simulink model "Lab05"  (R2024b)
settings: Solver=ode8  StartTime=0.0  StopTime=tf  FixedStep=0.025  RelTol=1e-3
values from neighbouring files (symbols this model uses):
  I = diag(Iv)    [initLab5.m]
  invI = inv(I)    [initLab5.m]
  w0 = [0.45; 0.52; 0.55]    [initLab5.m]
undefined symbols (not defined in the file or in its folder): IC
libraries: matrix_library x1
(part 1 of 4)
settings Model: Creator=elisa  LastModifiedBy=filippocamaleonte
settings ModelReferenceCC: ModelReferenceMinAlgLoopOccurrences=on
settings RTWCC: GPUComputeCapability=3.5

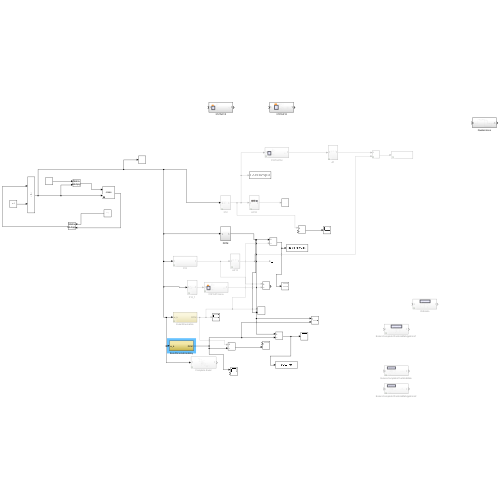
[thumbnail: Simulink's stored preview of the top-level diagram]
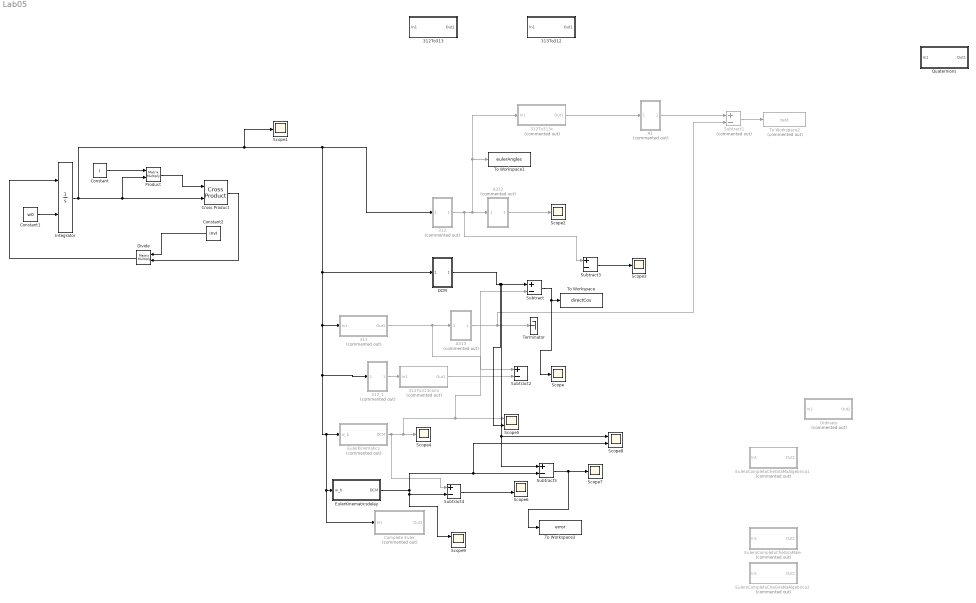
== system Lab05 ==
  312 : Subsystem  Commented=on
  312To313 : Subsystem
  312To313c : Subsystem  Commented=on
  312To313conv : Subsystem  Commented=on
  312_1 : Subsystem  Commented=on
  313 : Subsystem  Commented=on
  313To312 : Subsystem
  A1 : Subsystem  Commented=on
  A312 : Subsystem  Commented=on
  A313 : Subsystem  Commented=on
  Complete Euler : Subsystem  Commented=on
  Constant : Constant  Value=I
  Constant1 : Constant  Value=w0  VectorParams1D=off
  Constant2 : Constant  Value=invI
  Cross Product : matrix_library/Cross Product
  DCM : Subsystem
  Divide : Product  Inputs=**  Multiplication=Matrix(*)
  EulerKinematics : Subsystem  Commented=on
  EulerKinematicsdelay : Subsystem
  EuleroCompletoCheGiraMaAlgebrico1 : Subsystem  Commented=on
  EuleroCompletoCheGiraMaAlgebrico2 : Subsystem  Commented=on
  EuleroCompletoCheGiraMale : Subsystem  Commented=on
  Integrator : Integrator  InitialConditionSource=external
  Ordinato : Subsystem  Commented=on
  Product : Product  Multiplication=Matrix(*)
  Quaternions : Subsystem
  Scope{,1..4,7} (6 alike) : Scope
  Scope{5..6,8..9} (4 alike) : Scope  NumInputPorts=2
  Subtract{,2..5} (5 alike) : Sum  Inputs=+-
  Subtract1 : Sum  Commented=on  Inputs=+-
  Terminator : Terminator
  To Workspace : ToWorkspace  VariableName=directCos  SampleTime=-1
  To Workspace1 : ToWorkspace  VariableName=eulerAngles  SampleTime=-1
  To Workspace2 : ToWorkspace  Commented=on  VariableName=test  SampleTime=-1
  To Workspace3 : ToWorkspace  VariableName=error  SampleTime=-1
  wires:
  Product/1 -> Cross Product/1
  Cross Product/1 -> Divide/2
  Constant2/1 -> Divide/1
  Divide/1 -> Integrator/1
  Constant/1 -> Product/1
  Constant1/1 -> Integrator/2
  312/1(Out1) -> Subtract3/1, 312To313c/1(In1), To Workspace1/1, A312/1(In1)
  A313/1(Out1) -> Subtract1/2, Terminator/1
  Subtract/1 -> Scope/1, To Workspace/1
  A312/1(Out1) -> Scope2/1
  312To313c/1(Out1) -> A1/1(In1)
  A1/1(Out1) -> Subtract1/1
  Subtract1/1 -> To Workspace2/1
  312_1/1(Out1) -> 312To313conv/1(In1)
  312To313conv/1(Out1) -> Subtract2/2
  313/1(Out1) -> Subtract2/1, A313/1(In1)
  Subtract3/1 -> Scope3/1
  Integrator/1 -> Scope1/1, 313/1(In1), 312_1/1(In1), EulerKinematics/1(w_b), EulerKinematicsdelay/1(w_b), Complete Euler/1(In1), DCM/1(In1), 312/1(In1), Product/2, Cross Product/2
  EulerKinematics/1(DCM) -> Subtract4/1, Subtract/2, Scope5/1, Scope4/1
  DCM/1(Out1) -> Subtract/1, Scope8/1, Subtract5/1, Scope5/2
  Subtract4/1 -> Scope6/2
  EulerKinematicsdelay/1(DCM) -> Scope9/1, Subtract4/2, Scope8/2, Subtract5/2
  Subtract5/1 -> To Workspace3/1, Scope7/1

== system Lab05/312 ==
  In1 : Inport
  Cos1 : Trigonometry  Operator=cos
  Cos2 : Trigonometry  Operator=cos
  Demux : Demux  Outputs=3
  Divide1 : Product  Inputs=*/
  Integrator1 : Integrator  WrapState=on  WrappedStateUpperValue=2*pi  WrappedStateLowerValue=0
  Integrator2 : Integrator  InitialCondition=pi/4  WrapState=on
  Integrator3 : Integrator  WrapState=on  WrappedStateUpperValue=2*pi  WrappedStateLowerValue=0
  Mux : Mux  Inputs=3
  Product{1..7} (7 alike) : Product
  Sin : Trigonometry
  Subtract : Sum  Inputs=+-
  Subtract1 : Sum
  Subtract2 : Sum  Inputs=+-
  Subtract3 : Sum  Inputs=+-
  Tan : Trigonometry  Operator=tan
  Out1 : Outport
  wires:
  Product6/1 -> Subtract3/2
  Product5/1 -> Subtract3/1
  Product4/1 -> Subtract1/2
  Integrator3/1 -> [theta3]
  [wz] -> Product5/1
  Mux/1 -> Out1/1
  Product7/1 -> Subtract2/2
  Cos1/1 -> [cosPsi]
  [theta3] -> Sin/1, Cos1/1
  [cosPsi] -> Product1/2
  Demux/2 -> [wy]
  Tan/1 -> [tanThe]
  Product2/1 -> Subtract/2
  [wz] -> Product3/1
  [tanThe] -> Product7/2
  Cos2/1 -> [cosThe]
  [cosPsi] -> Product5/2
  Divide1/1 -> Integrator1/1
  Subtract1/1 -> Integrator2/1
  Demux/3 -> [wz]
  [theta1] -> Mux/1
  Subtract/1 -> Divide1/1
  Demux/1 -> [wx]
  Subtract2/1 -> Integrator3/1
  [theta2] -> Tan/1, Cos2/1
  [wy] -> Subtract2/1
  Integrator1/1 -> [theta1]
  Integrator2/1 -> [theta2]
  [wx] -> Product4/1
  [sinPsi] -> Product2/2
  In1/1 -> Demux/1
  Subtract3/1 -> Product7/1
  Product3/1 -> Subtract1/1
  [theta2] -> Mux/2
  [sinPsi] -> Product3/2
  [theta3] -> Mux/3
  [sinPsi] -> Product6/2
  [wx] -> Product6/1
  [wx] -> Product2/1
  [cosPsi] -> Product4/2
  [wz] -> Product1/1
  Product1/1 -> Subtract/1
  [cosThe] -> Divide1/2
  Sin/1 -> [sinPsi]

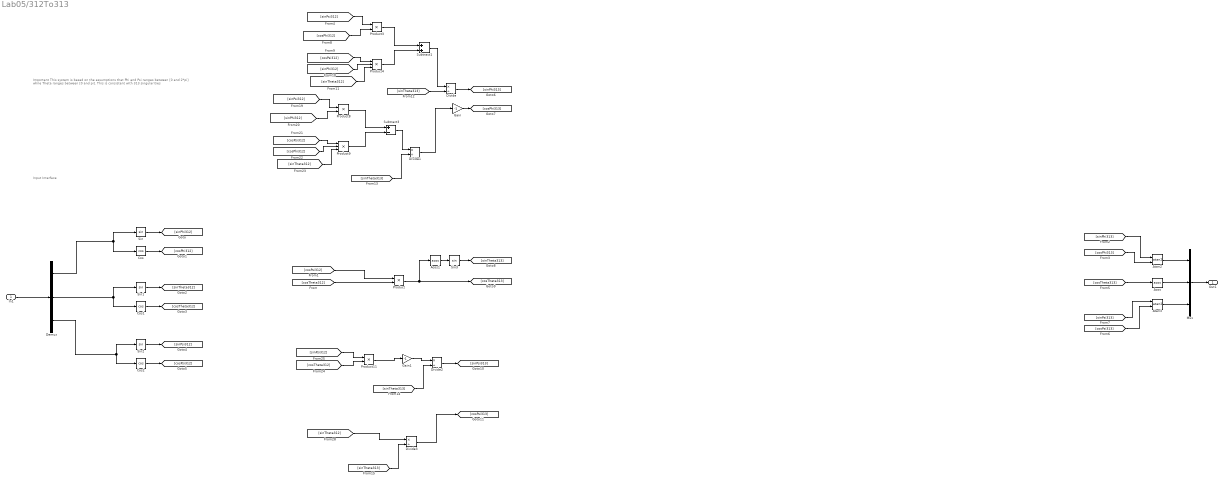
== system Lab05/312To313 ==
  note: Important
      |
      | This system is based on the assumptions that Phi and Psi ranges between [0 and 2*pi] while Theta ranges between [0 and pi]. This is consistent with 313 singularities
  note: Input Interface
  In1 : Inport
  Acos : Trigonometry  Operator=acos
  Acos1 : Trigonometry  Operator=acos
  Atan2 : Trigonometry  Operator=atan2
  Atan3 : Trigonometry  Operator=atan2
  Cos : Trigonometry  Operator=cos
  Cos1 : Trigonometry  Operator=cos
  Cos2 : Trigonometry  Operator=cos
  Demux : Demux  Outputs=3
  Divide{,1..3} (4 alike) : Product  Inputs=*/
  Gain : Gain  Gain=-1
  Gain1 : Gain  Gain=-1
  Mux : Mux  Inputs=3
  Product{,3,8,11} (4 alike) : Product
  Product4 : Product  Inputs=3
  Product9 : Product  Inputs=3
  Sin{,1..3} (4 alike) : Trigonometry
  Subtract1 : Sum
  Subtract3 : Sum  Inputs=+-
  Out1 : Outport
  wires:
  In1/1 -> Demux/1
  Mux/1 -> Out1/1
  Sin/1 -> [sinPhi312]
  Cos/1 -> [cosPhi312]
  Demux/1 -> Sin/1, Cos/1
  Sin1/1 -> [sinTheta312]
  Demux/2 -> Sin1/1, Cos1/1
  Cos1/1 -> [cosTheta312]
  Sin2/1 -> [sinPsi312]
  Cos2/1 -> [cosPsi312]
  Demux/3 -> Sin2/1, Cos2/1
  Product/1 -> Acos1/1, [cosTheta313]
  [cosTheta312] -> Product/2
  [cosPsi312] -> Product/1
  Atan2/1 -> Mux/1
  Acos/1 -> Mux/2
  Atan3/1 -> Mux/3
  [sinPhi313] -> Atan2/1
  [cosPhi313] -> Atan2/2
  [cosTheta313] -> Acos/1
  [cosPsi313] -> Atan3/2
  [sinPsi313] -> Atan3/1
  Sin3/1 -> [sinTheta313]
  Acos1/1 -> Sin3/1
  [cosPsi312] -> Product4/1
  [sinTheta312] -> Product4/3
  Product3/1 -> Subtract1/1
  [cosPhi312] -> Product3/2
  Product4/1 -> Subtract1/2
  [sinPsi312] -> Product3/1
  [sinPhi312] -> Product4/2
  Divide/1 -> [sinPhi313]
  [sinTheta313] -> Divide/2
  Subtract1/1 -> Divide/1
  Gain/1 -> [cosPhi313]
  Divide1/1 -> Gain/1
  [sinTheta313] -> Divide1/2
  [cosPsi312] -> Product9/1
  Product9/1 -> Subtract3/2
  Subtract3/1 -> Divide1/1
  [sinPsi312] -> Product8/1
  [cosPhi312] -> Product9/2
  [sinPhi312] -> Product8/2
  [sinTheta312] -> Product9/3
  Product8/1 -> Subtract3/1
  [sinTheta313] -> Divide2/2
  Divide2/1 -> [sinPsi313]
  [sinTheta313] -> Divide3/2
  Divide3/1 -> [cosPsi313]
  Product11/1 -> Gain1/1
  [sinPsi312] -> Product11/1
  [cosTheta312] -> Product11/2
  Gain1/1 -> Divide2/1
  [sinTheta312] -> Divide3/1

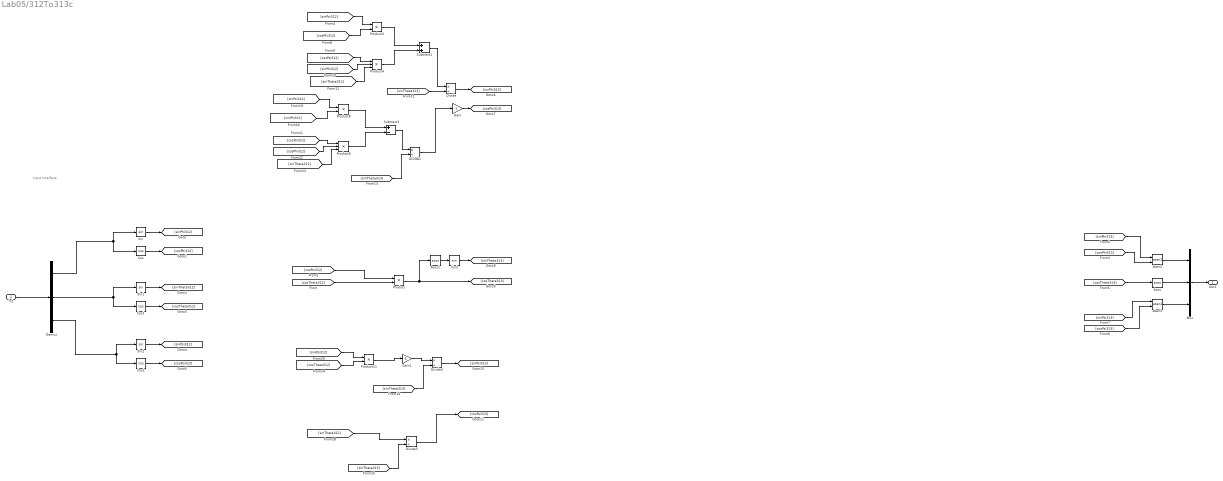
== system Lab05/312To313c ==
  note: Input Interface
  In1 : Inport
  Acos : Trigonometry  Operator=acos
  Acos1 : Trigonometry  Operator=acos
  Atan2 : Trigonometry  Operator=atan2
  Atan3 : Trigonometry  Operator=atan2
  Cos : Trigonometry  Operator=cos
  Cos1 : Trigonometry  Operator=cos
  Cos2 : Trigonometry  Operator=cos
  Demux : Demux  Outputs=3
  Divide{,1..3} (4 alike) : Product  Inputs=*/
  Gain : Gain  Gain=-1
  Gain1 : Gain  Gain=-1
  Mux : Mux  Inputs=3
  Product{,3,8,11} (4 alike) : Product
  Product4 : Product  Inputs=3
  Product9 : Product  Inputs=3
  Sin{,1..3} (4 alike) : Trigonometry
  Subtract1 : Sum
  Subtract3 : Sum  Inputs=+-
  Out1 : Outport
  wires:
  In1/1 -> Demux/1
  Mux/1 -> Out1/1
  Sin/1 -> [sinPhi312]
  Cos/1 -> [cosPhi312]
  Demux/1 -> Sin/1, Cos/1
  Sin1/1 -> [sinTheta312]
  Demux/2 -> Sin1/1, Cos1/1
  Cos1/1 -> [cosTheta312]
  Sin2/1 -> [sinPsi312]
  Cos2/1 -> [cosPsi312]
  Demux/3 -> Sin2/1, Cos2/1
  Product/1 -> Acos1/1, [cosTheta313]
  [cosTheta312] -> Product/2
  [cosPsi312] -> Product/1
  Atan2/1 -> Mux/1
  Acos/1 -> Mux/2
  Atan3/1 -> Mux/3
  [sinPhi313] -> Atan2/1
  [cosPhi313] -> Atan2/2
  [cosTheta313] -> Acos/1
  [cosPsi313] -> Atan3/2
  [sinPsi313] -> Atan3/1
  Sin3/1 -> [sinTheta313]
  Acos1/1 -> Sin3/1
  [cosPsi312] -> Product4/1
  [sinTheta312] -> Product4/3
  Product3/1 -> Subtract1/1
  [cosPhi312] -> Product3/2
  Product4/1 -> Subtract1/2
  [sinPsi312] -> Product3/1
  [sinPhi312] -> Product4/2
  Divide/1 -> [sinPhi313]
  [sinTheta313] -> Divide/2
  Subtract1/1 -> Divide/1
  Gain/1 -> [cosPhi313]
  Divide1/1 -> Gain/1
  [sinTheta313] -> Divide1/2
  [cosPsi312] -> Product9/1
  Product9/1 -> Subtract3/2
  Subtract3/1 -> Divide1/1
  [sinPsi312] -> Product8/1
  [cosPhi312] -> Product9/2
  [sinPhi312] -> Product8/2
  [sinTheta312] -> Product9/3
  Product8/1 -> Subtract3/1
  [sinTheta313] -> Divide2/2
  Divide2/1 -> [sinPsi313]
  [sinTheta313] -> Divide3/2
  Divide3/1 -> [cosPsi313]
  Product11/1 -> Gain1/1
  [sinPsi312] -> Product11/1
  [cosTheta312] -> Product11/2
  Gain1/1 -> Divide2/1
  [sinTheta312] -> Divide3/1

== system Lab05/312To313conv ==
  note: Important
      |
      | This system is based on the assumptions that Phi and Psi ranges between [0 and 2*pi] while Theta ranges between [0 and pi]. This is consistent with 313 singularities
  note: Input Interface
  In1 : Inport
  Acos : Trigonometry  Operator=acos
  Acos1 : Trigonometry  Operator=acos
  Atan2 : Trigonometry  Operator=atan2
  Atan3 : Trigonometry  Operator=atan2
  Cos : Trigonometry  Operator=cos
  Cos1 : Trigonometry  Operator=cos
  Cos2 : Trigonometry  Operator=cos
  Demux : Demux  Outputs=3
  Divide{,1..3} (4 alike) : Product  Inputs=*/
  Gain : Gain  Gain=-1
  Gain1 : Gain  Gain=-1
  Mux : Mux  Inputs=3
  Product{,3,8,11} (4 alike) : Product
  Product4 : Product  Inputs=3
  Product9 : Product  Inputs=3
  Sin{,1..3} (4 alike) : Trigonometry
  Subtract1 : Sum
  Subtract3 : Sum  Inputs=+-
  Out1 : Outport
  wires:
  In1/1 -> Demux/1
  Mux/1 -> Out1/1
  Sin/1 -> [sinPhi312]
  Cos/1 -> [cosPhi312]
  Demux/1 -> Sin/1, Cos/1
  Sin1/1 -> [sinTheta312]
  Demux/2 -> Sin1/1, Cos1/1
  Cos1/1 -> [cosTheta312]
  Sin2/1 -> [sinPsi312]
  Cos2/1 -> [cosPsi312]
  Demux/3 -> Sin2/1, Cos2/1
  Product/1 -> Acos1/1, [cosTheta313]
  [cosTheta312] -> Product/2
  [cosPsi312] -> Product/1
  Atan2/1 -> Mux/1
  Acos/1 -> Mux/2
  Atan3/1 -> Mux/3
  [sinPhi313] -> Atan2/1
  [cosPhi313] -> Atan2/2
  [cosTheta313] -> Acos/1
  [cosPsi313] -> Atan3/2
  [sinPsi313] -> Atan3/1
  Sin3/1 -> [sinTheta313]
  Acos1/1 -> Sin3/1
  [cosPsi312] -> Product4/1
  [sinTheta312] -> Product4/3
  Product3/1 -> Subtract1/1
  [cosPhi312] -> Product3/2
  Product4/1 -> Subtract1/2
  [sinPsi312] -> Product3/1
  [sinPhi312] -> Product4/2
  Divide/1 -> [sinPhi313]
  [sinTheta313] -> Divide/2
  Subtract1/1 -> Divide/1
  Gain/1 -> [cosPhi313]
  Divide1/1 -> Gain/1
  [sinTheta313] -> Divide1/2
  [cosPsi312] -> Product9/1
  Product9/1 -> Subtract3/2
  Subtract3/1 -> Divide1/1
  [sinPsi312] -> Product8/1
  [cosPhi312] -> Product9/2
  [sinPhi312] -> Product8/2
  [sinTheta312] -> Product9/3
  Product8/1 -> Subtract3/1
  [sinTheta313] -> Divide2/2
  Divide2/1 -> [sinPsi313]
  [sinTheta313] -> Divide3/2
  Divide3/1 -> [cosPsi313]
  Product11/1 -> Gain1/1
  [sinPsi312] -> Product11/1
  [cosTheta312] -> Product11/2
  Gain1/1 -> Divide2/1
  [sinTheta312] -> Divide3/1

== system Lab05/312_1 ==
  In1 : Inport
  Cos1 : Trigonometry  Operator=cos
  Cos2 : Trigonometry  Operator=cos
  Demux : Demux  Outputs=3
  Divide1 : Product  Inputs=*/
  Integrator1 : Integrator  WrapState=on  WrappedStateUpperValue=2*pi  WrappedStateLowerValue=0
  Integrator2 : Integrator  InitialCondition=pi/4  WrapState=on
  Integrator3 : Integrator  WrapState=on  WrappedStateUpperValue=2*pi  WrappedStateLowerValue=0
  Mux : Mux  Inputs=3
  Product{1..7} (7 alike) : Product
  Sin : Trigonometry
  Subtract : Sum  Inputs=+-
  Subtract1 : Sum
  Subtract2 : Sum  Inputs=+-
  Subtract3 : Sum  Inputs=+-
  Tan : Trigonometry  Operator=tan
  Out1 : Outport
  wires:
  Product6/1 -> Subtract3/2
  Product5/1 -> Subtract3/1
  Product4/1 -> Subtract1/2
  Integrator3/1 -> [theta3]
  [wz] -> Product5/1
  Mux/1 -> Out1/1
  Product7/1 -> Subtract2/2
  Cos1/1 -> [cosPsi]
  [theta3] -> Sin/1, Cos1/1
  [cosPsi] -> Product1/2
  Demux/2 -> [wy]
  Tan/1 -> [tanThe]
  Product2/1 -> Subtract/2
  [wz] -> Product3/1
  [tanThe] -> Product7/2
  Cos2/1 -> [cosThe]
  [cosPsi] -> Product5/2
  Divide1/1 -> Integrator1/1
  Subtract1/1 -> Integrator2/1
  Demux/3 -> [wz]
  [theta1] -> Mux/1
  Subtract/1 -> Divide1/1
  Demux/1 -> [wx]
  Subtract2/1 -> Integrator3/1
  [theta2] -> Tan/1, Cos2/1
  [wy] -> Subtract2/1
  Integrator1/1 -> [theta1]
  Integrator2/1 -> [theta2]
  [wx] -> Product4/1
  [sinPsi] -> Product2/2
  In1/1 -> Demux/1
  Subtract3/1 -> Product7/1
  Product3/1 -> Subtract1/1
  [theta2] -> Mux/2
  [sinPsi] -> Product3/2
  [theta3] -> Mux/3
  [sinPsi] -> Product6/2
  [wx] -> Product6/1
  [wx] -> Product2/1
  [cosPsi] -> Product4/2
  [wz] -> Product1/1
  Product1/1 -> Subtract/1
  [cosThe] -> Divide1/2
  Sin/1 -> [sinPsi]

== system Lab05/313 ==
  note: Phi
  note: Theta
  In1 : Inport
  Cos1 : Trigonometry  Operator=cos
  Cos2 : Trigonometry
  Demux : Demux  Outputs=3
  Divide : Product  Inputs=/
  Divide1 : Product  Inputs=*/
  Integrator1 : Integrator  WrapState=on  WrappedStateUpperValue=2*pi  WrappedStateLowerValue=0
  Integrator2 : Integrator  InitialCondition=pi/4  WrapState=on
  Integrator3 : Integrator  WrapState=on  WrappedStateUpperValue=2*pi  WrappedStateLowerValue=0
  Mux : Mux  Inputs=3
  Product{1..7} (7 alike) : Product
  Sin : Trigonometry
  Subtract : Sum
  Subtract1 : Sum  Inputs=-+
  Subtract2 : Sum  Inputs=+-
  Subtract3 : Sum
  Tan : Trigonometry  Operator=tan
  Out1 : Outport
  wires:
  [sinThe] -> Divide1/2
  Sin/1 -> [sinPsi]
  [wx] -> Product2/1
  [theta3] -> Mux/3
  [theta2] -> Mux/2
  Product3/1 -> Subtract1/1
  In1/1 -> Demux/1
  [sinPsi] -> Product3/2
  [sinPsi] -> Product6/2
  Subtract3/1 -> Product7/1
  Product1/1 -> Subtract/1
  [wx] -> Product6/1
  [wy] -> Product1/1
  [wz] -> Subtract2/1
  Subtract2/1 -> Integrator3/1
  [theta2] -> Tan/1, Cos2/1
  [cosPsi] -> Product4/2
  Demux/1 -> [wx]
  [sinPsi] -> Product2/2
  Integrator2/1 -> [theta2]
  [wx] -> Product4/1
  Tan/1 -> Divide/1
  [cosPsi] -> Product1/2
  Divide1/1 -> Integrator1/1
  Integrator1/1 -> [theta1]
  [ctanThe] -> Product7/2
  [cosPsi] -> Product5/2
  [wy] -> Product3/1
  Product2/1 -> Subtract/2
  Demux/2 -> [wy]
  Product5/1 -> Subtract3/1
  [wy] -> Product5/1
  Integrator3/1 -> [theta3]
  Product6/1 -> Subtract3/2
  Mux/1 -> Out1/1
  Product4/1 -> Subtract1/2
  [theta3] -> Sin/1, Cos1/1
  Product7/1 -> Subtract2/2
  Cos2/1 -> [sinThe]
  Subtract1/1 -> Integrator2/1
  [theta1] -> Mux/1
  Subtract/1 -> Divide1/1
  Demux/3 -> [wz]
  Cos1/1 -> [cosPsi]
  Divide/1 -> [ctanThe]

== system Lab05/313To312 ==
  note: Input Interface
  note: Important
      |
      | This system is based on the assumptions that Phi and Psi ranges between [0 and 2*pi] while Theta ranges between [-pi/2 and pi/2]. This is consistent with 312 singularities
  In1 : Inport
  Acos : Trigonometry  Operator=asin
  Acos1 : Trigonometry  Operator=asin
  Atan2 : Trigonometry  Operator=atan2
  Atan3 : Trigonometry  Operator=atan2
  Cos : Trigonometry  Operator=cos
  Cos1 : Trigonometry  Operator=cos
  Cos2 : Trigonometry  Operator=cos
  Demux : Demux  Outputs=3
  Divide{,1..3} (4 alike) : Product  Inputs=*/
  Gain : Gain  Gain=-1
  Gain1 : Gain  Gain=-1
  Mux : Mux  Inputs=3
  Product{,3,8,11} (4 alike) : Product
  Product4 : Product  Inputs=3
  Product9 : Product  Inputs=3
  Sin : Trigonometry
  Sin1 : Trigonometry
  Sin2 : Trigonometry
  Sin3 : Trigonometry  Operator=cos
  Subtract1 : Sum  Inputs=--
  Subtract3 : Sum  Inputs=-+
  Out1 : Outport
  wires:
  Cos/1 -> [cosPhi313]
  Sin/1 -> [sinPhi313]
  Cos1/1 -> [cosTheta313]
  Demux/3 -> Sin2/1, Cos2/1
  Demux/1 -> Sin/1, Cos/1
  Sin2/1 -> [sinPsi313]
  Sin1/1 -> [sinTheta313]
  In1/1 -> Demux/1
  Demux/2 -> Sin1/1, Cos1/1
  Cos2/1 -> [cosPsi313]
  Mux/1 -> Out1/1
  [sinTheta312] -> Acos/1
  Atan3/1 -> Mux/3
  Atan2/1 -> Mux/1
  [sinPhi312] -> Atan2/1
  [cosPhi312] -> Atan2/2
  [sinPsi312] -> Atan3/1
  [cosPsi312] -> Atan3/2
  Acos/1 -> Mux/2
  [sinTheta313] -> Product/2
  Product/1 -> Acos1/1, [sinTheta312]
  Sin3/1 -> [cosTheta312]
  [cosPsi313] -> Product/1
  Acos1/1 -> Sin3/1
  Gain/1 -> [sinPhi312]
  Divide/1 -> Gain/1
  [cosTheta312] -> Divide/2
  Product3/1 -> Subtract1/1
  [cosPhi313] -> Product3/2
  Product4/1 -> Subtract1/2
  [cosPsi313] -> Product4/1
  [sinPhi313] -> Product4/2
  Subtract1/1 -> Divide/1
  [sinPsi313] -> Product3/1
  [cosTheta313] -> Product4/3
  [cosTheta312] -> Divide1/2
  Divide1/1 -> [cosPhi312]
  [cosPsi313] -> Product9/1
  Product9/1 -> Subtract3/2
  [sinPsi313] -> Product8/1
  [sinPhi313] -> Product8/2
  Product8/1 -> Subtract3/1
  [cosTheta313] -> Product9/3
  Subtract3/1 -> Divide1/1
  [cosPhi313] -> Product9/2
  Divide2/1 -> Gain1/1
  [cosTheta312] -> Divide2/2
  Gain1/1 -> [sinPsi312]
  [sinTheta313] -> Product11/2
  Product11/1 -> Divide2/1
  [sinPsi313] -> Product11/1
  [cosTheta312] -> Divide3/2
  [cosTheta313] -> Divide3/1
  Divide3/1 -> [cosPsi312]

== system Lab05/A1 ==
  In1 : Inport
  Cos : Trigonometry  Operator=cos
  Cos1 : Trigonometry  Operator=cos
  Cos2 : Trigonometry  Operator=cos
  Demux : Demux  Outputs=3
  Gain : Gain  Gain=-1
  Matrix Concatenate : Concatenate  NumInputs=3  Mode=Multidimensional array
  Matrix Concatenate1 : Concatenate  NumInputs=3  Mode=Multidimensional array
  Matrix Concatenate3 : Concatenate  NumInputs=3  Mode=Multidimensional array  ConcatenateDimension=2
  Matrix Concatenate4 : Concatenate  NumInputs=3  Mode=Multidimensional array
  Product{1,3,5..6,8,10..12} (8 alike) : Product
  Product{2,4,7,9} (4 alike) : Product  Inputs=3
  Sin : Trigonometry
  Sin1 : Trigonometry
  Sin2 : Trigonometry
  Subtract : Sum  Inputs=+-
  Subtract1 : Sum  Inputs=--
  Subtract2 : Sum
  Subtract3 : Sum  Inputs=-+
  Out1 : Outport
  wires:
  In1/1 -> Demux/1
  [cosTheta] -> Product2/3
  Product7/1 -> Subtract2/2
  [sinTheta] -> Product11/2
  [sinPhi] -> Product8/2
  Sin/1 -> [sinPhi]
  [cosTheta] -> Product4/3
  [sinPhi] -> Product2/2
  [sinTheta] -> Product10/2
  Product5/1 -> Matrix Concatenate/3
  [cosPsi] -> Product6/1
  Demux/3 -> Sin2/1, Cos2/1
  Product9/1 -> Subtract3/2
  [cosTheta] -> Matrix Concatenate1/3
  Matrix Concatenate1/1 -> Matrix Concatenate3/3
  [sinPsi] -> Product11/1
  Product2/1 -> Subtract/2
  [sinPhi] -> Product4/2
  Subtract2/1 -> Matrix Concatenate4/1
  Matrix Concatenate4/1 -> Matrix Concatenate3/2
  [cosPsi] -> Product12/1
  Cos2/1 -> [cosPsi]
  Product10/1 -> Gain/1
  [sinPsi] -> Product2/1
  [sinPsi] -> Product8/1
  Sin2/1 -> [sinPsi]
  [cosTheta] -> Product7/3
  Subtract/1 -> Matrix Concatenate/1
  [cosPhi] -> Product10/1
  Subtract1/1 -> Matrix Concatenate/2
  Subtract3/1 -> Matrix Concatenate4/2
  Demux/2 -> Sin1/1, Cos1/1
  [cosTheta] -> Product9/3
  Product8/1 -> Subtract3/1
  [cosPhi] -> Product9/2
  [cosPsi] -> Product9/1
  Gain/1 -> Matrix Concatenate4/3
  [cosPsi] -> Product4/1
  Product11/1 -> Matrix Concatenate1/1
  Product1/1 -> Subtract/1
  [cosPhi] -> Product1/2
  [sinTheta] -> Product12/2
  [cosPhi] -> Product7/2
  [sinPhi] -> Product6/2
  Product6/1 -> Subtract2/1
  Demux/1 -> Sin/1, Cos/1
  [cosPsi] -> Product1/1
  [sinPsi] -> Product7/1
  Cos1/1 -> [cosTheta]
  Sin1/1 -> [sinTheta]
  [sinTheta] -> Product5/2
  [sinPsi] -> Product3/1
  Product12/1 -> Matrix Concatenate1/2
  [sinPhi] -> Product5/1
  Product3/1 -> Subtract1/1
  Product4/1 -> Subtract1/2
  [cosPhi] -> Product3/2
  Matrix Concatenate/1 -> Matrix Concatenate3/1
  Cos/1 -> [cosPhi]
  Matrix Concatenate3/1 -> Out1/1

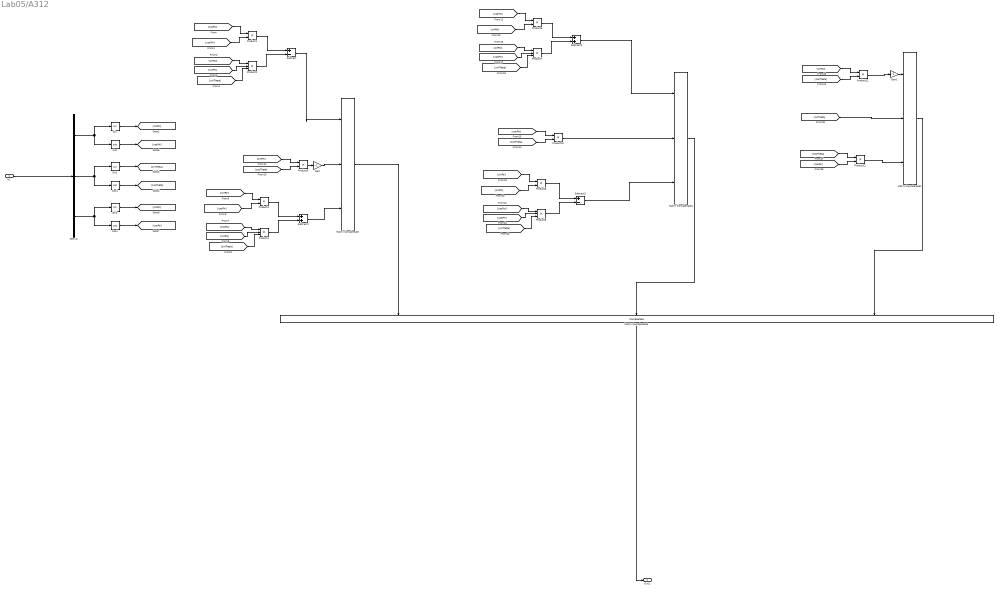
== system Lab05/A312 ==
  In1 : Inport
  Cos : Trigonometry  Operator=cos
  Cos1 : Trigonometry  Operator=cos
  Cos2 : Trigonometry  Operator=cos
  Demux : Demux  Outputs=3
  Gain : Gain  Gain=-1
  Gain1 : Gain  Gain=-1
  Matrix Concatenate : Concatenate  NumInputs=3  Mode=Multidimensional array
  Matrix Concatenate1 : Concatenate  NumInputs=3  Mode=Multidimensional array
  Matrix Concatenate3 : Concatenate  NumInputs=3  Mode=Multidimensional array  ConcatenateDimension=2
  Matrix Concatenate4 : Concatenate  NumInputs=3  Mode=Multidimensional array
  Product{1,3,5..6,8,10..12} (8 alike) : Product
  Product{2,4,7,9} (4 alike) : Product  Inputs=3
  Sin : Trigonometry
  Sin1 : Trigonometry
  Sin2 : Trigonometry
  Subtract : Sum  Inputs=+-
  Subtract1 : Sum
  Subtract2 : Sum
  Subtract3 : Sum  Inputs=+-
  Out1 : Outport
  wires:
  In1/1 -> Demux/1
  [sinTheta] -> Product2/3
  Product7/1 -> Subtract2/2
  [cosTheta] -> Product11/2
  [sinPhi] -> Product8/2
  Sin/1 -> [sinPhi]
  [sinPhi] -> Product2/2
  [cosTheta] -> Product10/2
  [cosPsi] -> Product6/1
  Demux/3 -> Sin2/1, Cos2/1
  Product9/1 -> Subtract3/2
  [sinTheta] -> Matrix Concatenate1/2
  Matrix Concatenate1/1 -> Matrix Concatenate3/3
  [sinPsi] -> Product11/1
  Product2/1 -> Subtract/2
  Subtract2/1 -> Matrix Concatenate4/1
  Matrix Concatenate4/1 -> Matrix Concatenate3/2
  [cosTheta] -> Product12/1
  Cos2/1 -> [cosPsi]
  [sinPsi] -> Product2/1
  [sinPsi] -> Product8/1
  Sin2/1 -> [sinPsi]
  [sinTheta] -> Product7/3
  Subtract/1 -> Matrix Concatenate/1
  [cosPhi] -> Product10/1
  Demux/2 -> Sin1/1, Cos1/1
  [sinTheta] -> Product9/3
  Product8/1 -> Subtract3/1
  [cosPhi] -> Product9/2
  [cosPsi] -> Product9/1
  Product11/1 -> Gain1/1
  Product1/1 -> Subtract/1
  [cosPhi] -> Product1/2
  [cosPsi] -> Product12/2
  [cosPhi] -> Product7/2
  [sinPhi] -> Product6/2
  Product6/1 -> Subtract2/1
  Demux/1 -> Sin/1, Cos/1
  [cosPsi] -> Product1/1
  [sinPsi] -> Product7/1
  Cos1/1 -> [cosTheta]
  Sin1/1 -> [sinTheta]
  Product12/1 -> Matrix Concatenate1/3
  Matrix Concatenate/1 -> Matrix Concatenate3/1
  Cos/1 -> [cosPhi]
  Matrix Concatenate3/1 -> Out1/1
  Gain1/1 -> Matrix Concatenate1/1
  Product10/1 -> Matrix Concatenate4/2
  Subtract3/1 -> Matrix Concatenate4/3
  [cosPsi] -> Product4/1
  Product4/1 -> Subtract1/2
  [cosPhi] -> Product3/2
  Product3/1 -> Subtract1/1
  [sinPsi] -> Product3/1
  [sinPhi] -> Product4/2
  [sinTheta] -> Product4/3
  [sinPhi] -> Product5/1
  [cosTheta] -> Product5/2
  Product5/1 -> Gain/1
  Subtract1/1 -> Matrix Concatenate/3
  Gain/1 -> Matrix Concatenate/2

== system Lab05/A313 ==
  In1 : Inport
  Cos : Trigonometry  Operator=cos
  Cos1 : Trigonometry  Operator=cos
  Cos2 : Trigonometry  Operator=cos
  Demux : Demux  Outputs=3
  Gain : Gain  Gain=-1
  Matrix Concatenate : Concatenate  NumInputs=3  Mode=Multidimensional array
  Matrix Concatenate1 : Concatenate  NumInputs=3  Mode=Multidimensional array
  Matrix Concatenate3 : Concatenate  NumInputs=3  Mode=Multidimensional array  ConcatenateDimension=2
  Matrix Concatenate4 : Concatenate  NumInputs=3  Mode=Multidimensional array
  Product{1,3,5..6,8,10..12} (8 alike) : Product
  Product{2,4,7,9} (4 alike) : Product  Inputs=3
  Sin : Trigonometry
  Sin1 : Trigonometry
  Sin2 : Trigonometry
  Subtract : Sum  Inputs=+-
  Subtract1 : Sum  Inputs=--
  Subtract2 : Sum
  Subtract3 : Sum  Inputs=-+
  Out1 : Outport
  wires:
  In1/1 -> Demux/1
  [cosTheta] -> Product2/3
  Product7/1 -> Subtract2/2
  [sinTheta] -> Product11/2
  [sinPhi] -> Product8/2
  Sin/1 -> [sinPhi]
  [cosTheta] -> Product4/3
  [sinPhi] -> Product2/2
  [sinTheta] -> Product10/2
  Product5/1 -> Matrix Concatenate/3
  [cosPsi] -> Product6/1
  Demux/3 -> Sin2/1, Cos2/1
  Product9/1 -> Subtract3/2
  [cosTheta] -> Matrix Concatenate1/3
  Matrix Concatenate1/1 -> Matrix Concatenate3/3
  [sinPsi] -> Product11/1
  Product2/1 -> Subtract/2
  [sinPhi] -> Product4/2
  Subtract2/1 -> Matrix Concatenate4/1
  Matrix Concatenate4/1 -> Matrix Concatenate3/2
  [cosPsi] -> Product12/1
  Cos2/1 -> [cosPsi]
  Product10/1 -> Gain/1
  [sinPsi] -> Product2/1
  [sinPsi] -> Product8/1
  Sin2/1 -> [sinPsi]
  [cosTheta] -> Product7/3
  Subtract/1 -> Matrix Concatenate/1
  [cosPhi] -> Product10/1
  Subtract1/1 -> Matrix Concatenate/2
  Subtract3/1 -> Matrix Concatenate4/2
  Demux/2 -> Sin1/1, Cos1/1
  [cosTheta] -> Product9/3
  Product8/1 -> Subtract3/1
  [cosPhi] -> Product9/2
  [cosPsi] -> Product9/1
  Gain/1 -> Matrix Concatenate4/3
  [cosPsi] -> Product4/1
  Product11/1 -> Matrix Concatenate1/1
  Product1/1 -> Subtract/1
  [cosPhi] -> Product1/2
  [sinTheta] -> Product12/2
  [cosPhi] -> Product7/2
  [sinPhi] -> Product6/2
  Product6/1 -> Subtract2/1
  Demux/1 -> Sin/1, Cos/1
  [cosPsi] -> Product1/1
  [sinPsi] -> Product7/1
  Cos1/1 -> [cosTheta]
  Sin1/1 -> [sinTheta]
  [sinTheta] -> Product5/2
  [sinPsi] -> Product3/1
  Product12/1 -> Matrix Concatenate1/2
  [sinPhi] -> Product5/1
  Product3/1 -> Subtract1/1
  Product4/1 -> Subtract1/2
  [cosPhi] -> Product3/2
  Matrix Concatenate/1 -> Matrix Concatenate3/1
  Cos/1 -> [cosPhi]
  Matrix Concatenate3/1 -> Out1/1

== system Lab05/Complete Euler ==
  In1 : Inport
  312 : Subsystem
  312To313 : Subsystem
  313 : Subsystem
  313To312 : Subsystem
  A312 : Subsystem
  A313 : Subsystem
  Abs : Abs  SaturateOnIntegerOverflow=off
  Abs1 : Abs  SaturateOnIntegerOverflow=off
  Constant : Constant
  Constant1 : Constant  Value=0
  Constant2 : Constant  Value=0
  Constant3 : Constant
  Cos : Trigonometry  Operator=cos
  Gain : Gain  Gain=-1
  Gain1 : Gain  Gain=-1
  Merge : Merge
  Selector : Selector  InputPortWidth=3  IndexOptions=Index vector (dialog)  Indices=[2]  OutputSizes=1
  Selector1 : Selector  InputPortWidth=3  IndexOptions=Index vector (dialog)  Indices=[2]  OutputSizes=1
  Sin : Trigonometry
  Switch : Switch  Criteria=u2 > Threshold  Threshold=-0.0001  SaturateOnIntegerOverflow=off  InputSameDT=off
  Switch1 : Switch  Criteria=u2 > Threshold  Threshold=-0.001  SaturateOnIntegerOverflow=off  InputSameDT=off
  Out1 : Outport
  wires:
  312To313/1(Out1) -> 313/2(In2)
  In1/1 -> 313/1(In1), 312/1(In1)
  313/1(Out1) -> 313To312/1(In1), Selector1/1, A313/1(In1)
  312/1(Out1) -> Selector/1, 312To313/1(In1), A312/1(In1)
  A313/1(Out1) -> Merge/2
  A312/1(Out1) -> Merge/1
  313To312/1(Out1) -> 312/2(In2)
  Selector/1 -> Cos/1
  Merge/1 -> Out1/1
  Cos/1 -> Abs/1
  Sin/1 -> Abs1/1
  Selector1/1 -> Sin/1
  Switch/1 -> 312/Enable
  Abs/1 -> Gain/1
  Switch1/1 -> 313/Enable
  Abs1/1 -> Gain1/1
  Constant/1 -> Switch1/1
  Gain/1 -> Switch1/2
  Gain1/1 -> Switch/2
  Constant1/1 -> Switch1/3
  Constant2/1 -> Switch/3
  Constant3/1 -> Switch/1

== system Lab05/DCM ==
  In1 : Inport
  A312 : Subsystem
  Constant3 : Constant  Value=IC.angles
  Gain : Gain  Gain=-1
  Integrator1 : Integrator  InitialConditionSource=external
  Product1 : Product  Multiplication=Matrix(*)
  Subsystem : Subsystem
  Subsystem1 : Subsystem
  w^ : Subsystem
  Out1 : Outport
  wires:
  w^/1(Out1) -> Gain/1
  Gain/1 -> Product1/1
  In1/1 -> w^/1(In1)
  Product1/1 -> Integrator1/1
  Constant3/1 -> A312/1(In1)
  Integrator1/1 -> Subsystem/1(In1)
  Subsystem/1(Out1) -> Subsystem1/1(In1)
  A312/1(Out1) -> Integrator1/2
  Subsystem1/1(Out1) -> Product1/2, Out1/1

== system Lab05/EulerKinematics ==
  note: Logic
  note: The flag is set to -1 when 313 is used and to 1 when 312 is used
  w_b : Inport
  312 Propagator : Subsystem
  312To313 : Subsystem
  313 Propagator : Subsystem
  313To312 : Subsystem
  A312 : Subsystem
  A313 : Subsystem
  Abs : Abs  SaturateOnIntegerOverflow=off
  Cos : Trigonometry  Operator=cos
  IC : InitialCondition  Value=IC.angles
  IC1 : InitialCondition  Value=IC.angles
  IC3 : InitialCondition
  Relay : Relay  OnSwitchValue=0.85  OffSwitchValue=0.15  OffOutputValue=-1
  Selector1 : Selector  InputPortWidth=3  IndexOptions=Index vector (dialog)  Indices=[2]  OutputSizes=1
  Switch : Switch  Criteria=u2 > Threshold  SaturateOnIntegerOverflow=off  InputSameDT=off
  Switch1 : Switch  Criteria=u2 > Threshold  SaturateOnIntegerOverflow=off  InputSameDT=off
  To Workspace : ToWorkspace  VariableName=flag  SampleTime=-1
  DCM : Outport
  wires:
  [EulerFlag] -> Switch1/2
  Cos/1 -> Abs/1
  Selector1/1 -> Cos/1
  Abs/1 -> Relay/1
  A313/1(Out1) -> Switch/3
  [Euler313] -> Switch1/3
  w_b/1 -> 313 Propagator/2(w_b), 312 Propagator/2(w_b)  "w_b"
  313 Propagator/1(EA) -> A313/1(Euler Angles), [Euler313]  "EulerAngles313"
  [Euler312] -> Switch1/1
  A312/1(DCM) -> Switch/1
  Switch1/1 -> Selector1/1
  Switch/1 -> DCM/1  "DCM"
  Relay/1 -> IC3/1
  IC3/1 -> To Workspace/1, [EulerFlag]
  313To312/1(Out1) -> IC1/1
  312To313/1(Out1) -> IC/1
  [Euler313] -> 313To312/1(In1)
  IC1/1 -> 312 Propagator/1(IC)
  IC/1 -> 313 Propagator/3(IC)
  [Euler312] -> 312To313/1(In1)
  [EulerFlag] -> Switch/2, 312 Propagator/3(Reset), 313 Propagator/1(Reset)
  312 Propagator/1(EA) -> [Euler312], A312/1(Euler Angles)  "EulerAngles312"

== system Lab05/EulerKinematicsdelay ==
  note: Logic
  note: The flag is set to -1 when 313 is used and to 1 when 312 is used
  w_b : Inport
  312 Propagator : Subsystem
  312To313 : Subsystem
  313 Propagator : Subsystem
  313To312 : Subsystem
  A312 : Subsystem
  A313 : Subsystem
  Abs : Abs  SaturateOnIntegerOverflow=off
  Cos : Trigonometry  Operator=cos
  IC : InitialCondition  Value=IC.angles
  IC1 : InitialCondition  Value=IC.angles
  IC3 : InitialCondition
  Relay : Relay  OnSwitchValue=0.75  OffSwitchValue=0.35  OffOutputValue=-1
  Selector1 : Selector  InputPortWidth=3  IndexOptions=Index vector (dialog)  Indices=[2]  OutputSizes=1
  Switch : Switch  Criteria=u2 > Threshold  SaturateOnIntegerOverflow=off  InputSameDT=off
  Switch1 : Switch  Criteria=u2 > Threshold  SaturateOnIntegerOverflow=off  InputSameDT=off
  To Workspace : ToWorkspace  VariableName=flag1  SampleTime=-1
  To Workspace1 : ToWorkspace  VariableName=eu312  SampleTime=-1
  To Workspace2 : ToWorkspace  VariableName=eu313  SampleTime=-1
  DCM : Outport
  wires:
  Cos/1 -> Abs/1
  Selector1/1 -> Cos/1
  Abs/1 -> Relay/1
  A313/1(Out1) -> Switch/3
  w_b/1 -> 313 Propagator/2(w_b), 312 Propagator/2(w_b)  "w_b"
  313 Propagator/1(EA) -> [Euler313], A313/1(Euler Angles)  "EulerAngles313"
  A312/1(DCM) -> Switch/1
  Switch1/1 -> Selector1/1
  Switch/1 -> DCM/1  "DCM"
  313To312/1(Out1) -> IC1/1
  312To313/1(Out1) -> IC/1
  IC1/1 -> 312 Propagator/1(IC)
  IC/1 -> 313 Propagator/3(IC)
  [EulerFlag] -> Switch/2, 312 Propagator/3(Reset), 313 Propagator/1(Reset)
  312 Propagator/1(EA) -> [Euler312], A312/1(Euler Angles)  "EulerAngles312"
  312 Propagator/2(Out1) -> 312To313/1(In1)
  313 Propagator/2(Out1) -> 313To312/1(In1)
  Relay/1 -> IC3/1
  [Euler312] -> To Workspace1/1, Switch1/1
  [Euler313] -> To Workspace2/1, Switch1/3
  [EulerFlag] -> Switch1/2
  IC3/1 -> To Workspace/1, [EulerFlag]

== system Lab05/EuleroCompletoCheGiraMaAlgebrico1 ==
  note: Logic
  note: The flag is set to -1 when 313 is used and to 1 when 312 is used
  In1 : Inport
  312 : Subsystem
  312To313 : Subsystem
  313 : Subsystem
  313To312 : Subsystem
  A312 : Subsystem
  A313 : Subsystem
  Abs : Abs  SaturateOnIntegerOverflow=off
  Cos : Trigonometry  Operator=cos
  IC : InitialCondition  Value=IC.angles
  IC1 : InitialCondition  Value=IC.angles
  IC3 : InitialCondition
  Relay : Relay  OnSwitchValue=0.7  OffSwitchValue=0.2  OffOutputValue=-1
  Selector1 : Selector  InputPortWidth=3  IndexOptions=Index vector (dialog)  Indices=[2]  OutputSizes=1
  Switch : Switch  Criteria=u2 > Threshold  SaturateOnIntegerOverflow=off  InputSameDT=off
  Switch1 : Switch  Criteria=u2 > Threshold  SaturateOnIntegerOverflow=off  InputSameDT=off
  To Workspace : ToWorkspace  VariableName=flag  SampleTime=-1
  Out1 : Outport
  wires:
  Switch/1 -> Out1/1
  Abs/1 -> Relay/1
  Cos/1 -> Abs/1
  [EulerFlag] -> 312/3(In3), Switch/2, 313/1(In3)
  A312/1(Out1) -> Switch/1
  A313/1(Out1) -> Switch/3
  Switch1/1 -> Selector1/1
  In1/1 -> 313/2(In1), 312/2(In1)
  [Euler313] -> Switch1/3
  [Euler312] -> Switch1/1
  Selector1/1 -> Cos/1
  [EulerFlag] -> Switch1/2
  IC3/1 -> To Workspace/1, [EulerFlag]
  Relay/1 -> IC3/1
  [Euler313] -> 313To312/1(In1)
  312/1(Out1) -> A312/1(In1), [Euler312]
  313/1(Out1) -> A313/1(In1), [Euler313]
  [Euler312] -> IC/1
  313To312/1(Out1) -> IC1/1
  312To313/1(Out1) -> 313/3(In2)
  IC/1 -> 312To313/1(In1)
  IC1/1 -> 312/1(In2)

== system Lab05/EuleroCompletoCheGiraMaAlgebrico2 ==
  note: Logic
  note: The flag is set to -1 when 313 is used and to 1 when 312 is used
  In1 : Inport
  312 : Subsystem
  312To313 : Subsystem
  313 : Subsystem
  313To1 : Subsystem
  313To312 : Subsystem
  A312 : Subsystem
  A313 : Subsystem
  Abs : Abs  SaturateOnIntegerOverflow=off
  Cos : Trigonometry  Operator=cos
  Gain : Gain  Gain=-1
  IC3 : InitialCondition
  Relay : Relay  OnSwitchValue=0.8  OffSwitchValue=0.2  OffOutputValue=-1
  Scope : Scope
  Scope1 : Scope
  Scope2 : Scope
  Selector1 : Selector  InputPortWidth=3  IndexOptions=Index vector (dialog)  Indices=[2]  OutputSizes=1
  Subtract : Sum  Inputs=+-
  Subtract1 : Sum  Inputs=+-
  Switch : Switch  Criteria=u2 > Threshold  SaturateOnIntegerOverflow=off  InputSameDT=off
  Switch1 : Switch  Criteria=u2 > Threshold  SaturateOnIntegerOverflow=off  InputSameDT=off
  To Workspace : ToWorkspace  VariableName=flag  SampleTime=-1
  Out1 : Outport
  wires:
  Switch/1 -> Out1/1
  Abs/1 -> Relay/1
  Cos/1 -> Abs/1
  [EulerFlag] -> Gain/1, Switch/2, 313/3(In3)
  A312/1(Out1) -> Switch/1, Scope2/1, Subtract1/1
  A313/1(Out1) -> Subtract1/2, Switch/3
  Switch1/1 -> Selector1/1
  In1/1 -> 313/2(In1), 312/1(In1)
  [EulerFlag] -> 312/3(In3)
  313To312/1(Out1) -> 312/2(In2)
  312To313/1(Out1) -> 313/1(In2)
  [Euler313] -> Switch1/3
  [Euler312] -> Switch1/1
  Selector1/1 -> Cos/1
  [EulerFlag] -> Switch1/2
  IC3/1 -> To Workspace/1, [EulerFlag]
  [Euler312] -> Subtract/2
  Subtract/1 -> Scope/1
  Relay/1 -> IC3/1
  [Euler313] -> 313To1/1(In1)
  313To1/1(Out1) -> Subtract/1
  Subtract1/1 -> Scope1/1
  [Euler312] -> 312To313/1(In1)
  [Euler313] -> 313To312/1(In1)
  312/1(Out1) -> [Euler312], A312/1(In1)
  313/1(Out1) -> A313/1(In1), [Euler313]

== system Lab05/EuleroCompletoCheGiraMale ==
  note: Logic
  note: The flag is set to -1 when 313 is used and to 1 when 312 is used
  In1 : Inport
  312 : Subsystem
  312To313 : Subsystem
  313 : Subsystem
  313To1 : Subsystem
  313To312 : Subsystem
  A312 : Subsystem
  A313 : Subsystem
  Abs : Abs  SaturateOnIntegerOverflow=off
  Cos : Trigonometry  Operator=cos
  Gain : Gain  Gain=-1
  IC : InitialCondition
  IC1 : InitialCondition  Value=IC.angles
  IC2 : InitialCondition  Value=IC.angles
  IC3 : InitialCondition
  Relay : Relay  OnSwitchValue=0.80  OffSwitchValue=0.2  OffOutputValue=-1
  Scope : Scope
  Scope1 : Scope
  Selector1 : Selector  InputPortWidth=3  IndexOptions=Index vector (dialog)  Indices=[2]  OutputSizes=1
  Subtract : Sum  Inputs=+-
  Subtract1 : Sum  Inputs=+-
  Switch : Switch  Criteria=u2 > Threshold  SaturateOnIntegerOverflow=off  InputSameDT=off
  Switch1 : Switch  Criteria=u2 > Threshold  SaturateOnIntegerOverflow=off  InputSameDT=off
  To Workspace : ToWorkspace  VariableName=flag  SaveFormat=Timeseries  SampleTime=-1
  Unit Delay : UnitDelay  SampleTime=-1  HasFrameUpgradeWarning=on
  Unit Delay1 : UnitDelay  SampleTime=-1  HasFrameUpgradeWarning=on
  Unit Delay2 : UnitDelay  SampleTime=-1  HasFrameUpgradeWarning=on
  Out1 : Outport
  wires:
  Switch/1 -> Out1/1
  Abs/1 -> Relay/1
  Cos/1 -> Abs/1
  [EulerFlag] -> Gain/1, Switch/2
  312/1(Out1) -> IC2/1
  A312/1(Out1) -> Subtract1/1, Switch/1
  313/1(Out1) -> IC1/1
  A313/1(Out1) -> Subtract1/2, Switch/3
  Switch1/1 -> Selector1/1
  [EulerFlag] -> IC/1
  In1/1 -> 313/2(In1), 312/1(In1)
  [EulerFlag] -> 312/Enable
  Gain/1 -> 313/Enable
  313To312/1(Out1) -> 312/2(In2)
  312To313/1(Out1) -> 313/1(In2)
  [Euler312] -> Unit Delay2/1
  [Euler313] -> Unit Delay1/1
  [Euler313] -> Switch1/3
  [Euler312] -> Switch1/1
  Selector1/1 -> Cos/1
  IC1/1 -> A313/1(In1), [Euler313]
  IC2/1 -> [Euler312], A312/1(In1)
  IC/1 -> Switch1/2
  IC3/1 -> To Workspace/1, [EulerFlag]
  [Euler312] -> Subtract/2
  Subtract/1 -> Scope/1
  Unit Delay/1 -> IC3/1
  Relay/1 -> Unit Delay/1
  Unit Delay1/1 -> 313To312/1(In1)
  [Euler313] -> 313To1/1(In1)
  313To1/1(Out1) -> Subtract/1
  Subtract1/1 -> Scope1/1
  Unit Delay2/1 -> 312To313/1(In1)

== system Lab05/Ordinato ==
  note: Logic
  note: The flag is set to -1 when 313 is used and to 1 when 312 is used
  In2 : Inport
  312 : Subsystem
  312To313 : Subsystem
  313 : Subsystem
  313To312 : Subsystem
  A312 : Subsystem
  A313 : Subsystem
  Abs : Abs  SaturateOnIntegerOverflow=off
  Cos : Trigonometry  Operator=cos
  IC : InitialCondition  Value=IC.angles
  IC1 : InitialCondition  Value=IC.angles
  IC3 : InitialCondition
  Relay : Relay  OnSwitchValue=0.65  OffSwitchValue=0.35  OffOutputValue=-1
  Selector1 : Selector  InputPortWidth=3  IndexOptions=Index vector (dialog)  Indices=[2]  OutputSizes=1
  Switch : Switch  Criteria=u2 > Threshold  SaturateOnIntegerOverflow=off  InputSameDT=off
  Switch1 : Switch  Criteria=u2 > Threshold  SaturateOnIntegerOverflow=off  InputSameDT=off
  To Workspace : ToWorkspace  VariableName=flag  SampleTime=-1
  Out2 : Outport
  wires:
  [EulerFlag] -> Switch1/2
  Cos/1 -> Abs/1
  Selector1/1 -> Cos/1
  Abs/1 -> Relay/1
  A313/1(Out1) -> Switch/3
  [Euler313] -> Switch1/3
  In2/1 -> 313/2(In1), 312/2(In1)
  313/1(Out1) -> A313/1(In1), [Euler313]
  [Euler312] -> Switch1/1
  A312/1(Out1) -> Switch/1
  Switch1/1 -> Selector1/1
  Switch/1 -> Out2/1
  Relay/1 -> IC3/1
  IC3/1 -> To Workspace/1, [EulerFlag]
  313To312/1(Out1) -> IC1/1
  312To313/1(Out1) -> IC/1
  [Euler313] -> 313To312/1(In1)
  IC1/1 -> 312/1(In2)
  IC/1 -> 313/3(In2)
  [Euler312] -> 312To313/1(In1)
  [EulerFlag] -> Switch/2, 312/3(In3), 313/1(In3)
  312/1(Out1) -> [Euler312], A312/1(In1)

== system Lab05/Quaternions ==
  In1 : Inport
  Gain : Gain  Gain=0.5  Multiplication=Matrix(u*K)
  Integrator : Integrator
  Matrix Multiply : Product  Multiplication=Matrix(*)
  Omega : Subsystem
  Out1 : Outport
  wires:
  Integrator/1 -> Matrix Multiply/2, Out1/1
  In1/1 -> Omega/1(In1)
  Omega/1(Out1) -> Gain/1
  Gain/1 -> Matrix Multiply/1
  Matrix Multiply/1 -> Integrator/1

== system Lab05/Complete Euler/312 ==
  In1 : Inport
  In2 : Inport  Port=2
  Enable : EnablePort  StatesWhenEnabling=reset
  Cos1 : Trigonometry  Operator=cos
  Cos2 : Trigonometry  Operator=cos
  Demux : Demux  Outputs=3
  Demux1 : Demux  Outputs=3
  Divide1 : Product  Inputs=*/
  IC : InitialCondition  Value=IC.angles
  Integrator1 : Integrator  InitialConditionSource=external  WrapState=on  WrappedStateUpperValue=2*pi  WrappedStateLowerValue=0
  Integrator2 : Integrator  InitialConditionSource=external  WrapState=on
  Integrator3 : Integrator  InitialConditionSource=external  WrapState=on  WrappedStateUpperValue=2*pi  WrappedStateLowerValue=0
  Mux : Mux  Inputs=3
  Product{1..7} (7 alike) : Product
  Sin : Trigonometry
  Subtract : Sum  Inputs=+-
  Subtract1 : Sum
  Subtract2 : Sum  Inputs=+-
  Subtract3 : Sum  Inputs=+-
  Tan : Trigonometry  Operator=tan
  Out1 : Outport
  wires:
  Product6/1 -> Subtract3/2
  Product5/1 -> Subtract3/1
  Product4/1 -> Subtract1/2
  Integrator3/1 -> [theta3]
  [wz] -> Product5/1
  Mux/1 -> Out1/1
  Product7/1 -> Subtract2/2
  Cos1/1 -> [cosPsi]
  [theta3] -> Sin/1, Cos1/1
  [cosPsi] -> Product1/2
  Demux/2 -> [wy]
  Tan/1 -> [tanThe]
  Product2/1 -> Subtract/2
  [wz] -> Product3/1
  [tanThe] -> Product7/2
  Cos2/1 -> [cosThe]
  [cosPsi] -> Product5/2
  Divide1/1 -> Integrator1/1
  Subtract1/1 -> Integrator2/1
  Demux/3 -> [wz]
  [theta1] -> Mux/1
  Subtract/1 -> Divide1/1
  Demux/1 -> [wx]
  Subtract2/1 -> Integrator3/1
  [theta2] -> Tan/1, Cos2/1
  [wy] -> Subtract2/1
  Integrator1/1 -> [theta1]
  Integrator2/1 -> [theta2]
  [wx] -> Product4/1
  [sinPsi] -> Product2/2
  In1/1 -> Demux/1
  Subtract3/1 -> Product7/1
  Product3/1 -> Subtract1/1
  [theta2] -> Mux/2
  [sinPsi] -> Product3/2
  [theta3] -> Mux/3
  [sinPsi] -> Product6/2
  [wx] -> Product6/1
  [wx] -> Product2/1
  [cosPsi] -> Product4/2
  [wz] -> Product1/1
  Product1/1 -> Subtract/1
  [cosThe] -> Divide1/2
  Sin/1 -> [sinPsi]
  Demux1/1 -> Integrator1/2
  Demux1/2 -> Integrator2/2
  Demux1/3 -> Integrator3/2
  In2/1 -> IC/1
  IC/1 -> Demux1/1

== system Lab05/Complete Euler/312To313 ==
  note: Important
      |
      | This system is based on the assumptions that Phi and Psi ranges between [0 and 2*pi] while Theta ranges between [0 and pi]. This is consistent with 313 singularities
  note: Input Interface
  In1 : Inport
  Acos : Trigonometry  Operator=acos
  Acos1 : Trigonometry  Operator=acos
  Atan2 : Trigonometry  Operator=atan2
  Atan3 : Trigonometry  Operator=atan2
  Cos : Trigonometry  Operator=cos
  Cos1 : Trigonometry  Operator=cos
  Cos2 : Trigonometry  Operator=cos
  Demux : Demux  Outputs=3
  Divide{,1..3} (4 alike) : Product  Inputs=*/
  Gain : Gain  Gain=-1
  Gain1 : Gain  Gain=-1
  Mux : Mux  Inputs=3
  Product{,3,8,11} (4 alike) : Product
  Product4 : Product  Inputs=3
  Product9 : Product  Inputs=3
  Sin{,1..3} (4 alike) : Trigonometry
  Subtract1 : Sum
  Subtract3 : Sum  Inputs=+-
  Out1 : Outport
  wires:
  In1/1 -> Demux/1
  Mux/1 -> Out1/1
  Sin/1 -> [sinPhi312]
  Cos/1 -> [cosPhi312]
  Demux/1 -> Sin/1, Cos/1
  Sin1/1 -> [sinTheta312]
  Demux/2 -> Sin1/1, Cos1/1
  Cos1/1 -> [cosTheta312]
  Sin2/1 -> [sinPsi312]
  Cos2/1 -> [cosPsi312]
  Demux/3 -> Sin2/1, Cos2/1
  Product/1 -> Acos1/1, [cosTheta313]
  [cosTheta312] -> Product/2
  [cosPsi312] -> Product/1
  Atan2/1 -> Mux/1
  Acos/1 -> Mux/2
  Atan3/1 -> Mux/3
  [sinPhi313] -> Atan2/1
  [cosPhi313] -> Atan2/2
  [cosTheta313] -> Acos/1
  [cosPsi313] -> Atan3/2
  [sinPsi313] -> Atan3/1
  Sin3/1 -> [sinTheta313]
  Acos1/1 -> Sin3/1
  [cosPsi312] -> Product4/1
  [sinTheta312] -> Product4/3
  Product3/1 -> Subtract1/1
  [cosPhi312] -> Product3/2
  Product4/1 -> Subtract1/2
  [sinPsi312] -> Product3/1
  [sinPhi312] -> Product4/2
  Divide/1 -> [sinPhi313]
  [sinTheta313] -> Divide/2
  Subtract1/1 -> Divide/1
  Gain/1 -> [cosPhi313]
  Divide1/1 -> Gain/1
  [sinTheta313] -> Divide1/2
  [cosPsi312] -> Product9/1
  Product9/1 -> Subtract3/2
  Subtract3/1 -> Divide1/1
  [sinPsi312] -> Product8/1
  [cosPhi312] -> Product9/2
  [sinPhi312] -> Product8/2
  [sinTheta312] -> Product9/3
  Product8/1 -> Subtract3/1
  [sinTheta313] -> Divide2/2
  Divide2/1 -> [sinPsi313]
  [sinTheta313] -> Divide3/2
  Divide3/1 -> [cosPsi313]
  Product11/1 -> Gain1/1
  [sinPsi312] -> Product11/1
  [cosTheta312] -> Product11/2
  Gain1/1 -> Divide2/1
  [sinTheta312] -> Divide3/1

== system Lab05/Complete Euler/313 ==
  note: Phi
  note: Theta
  In1 : Inport
  In2 : Inport  Port=2
  Enable : EnablePort  StatesWhenEnabling=reset
  Cos1 : Trigonometry  Operator=cos
  Cos2 : Trigonometry
  Demux : Demux  Outputs=3
  Demux1 : Demux  Outputs=3
  Divide : Product  Inputs=/
  Divide1 : Product  Inputs=*/
  IC : InitialCondition  Value=IC.angles
  Integrator1 : Integrator  InitialConditionSource=external  WrapState=on  WrappedStateUpperValue=2*pi  WrappedStateLowerValue=0
  Integrator2 : Integrator  InitialConditionSource=external  InitialCondition=pi/4  WrapState=on
  Integrator3 : Integrator  InitialConditionSource=external  WrapState=on  WrappedStateUpperValue=2*pi  WrappedStateLowerValue=0
  Mux : Mux  Inputs=3
  Product{1..7} (7 alike) : Product
  Sin : Trigonometry
  Subtract : Sum
  Subtract1 : Sum  Inputs=-+
  Subtract2 : Sum  Inputs=+-
  Subtract3 : Sum
  Tan : Trigonometry  Operator=tan
  Out1 : Outport
  wires:
  [sinThe] -> Divide1/2
  Sin/1 -> [sinPsi]
  [wx] -> Product2/1
  [theta3] -> Mux/3
  [theta2] -> Mux/2
  Product3/1 -> Subtract1/1
  In1/1 -> Demux/1
  [sinPsi] -> Product3/2
  [sinPsi] -> Product6/2
  Subtract3/1 -> Product7/1
  Product1/1 -> Subtract/1
  [wx] -> Product6/1
  [wy] -> Product1/1
  [wz] -> Subtract2/1
  Subtract2/1 -> Integrator3/1
  [theta2] -> Tan/1, Cos2/1
  [cosPsi] -> Product4/2
  Demux/1 -> [wx]
  [sinPsi] -> Product2/2
  Integrator2/1 -> [theta2]
  [wx] -> Product4/1
  Tan/1 -> Divide/1
  [cosPsi] -> Product1/2
  Divide1/1 -> Integrator1/1
  Integrator1/1 -> [theta1]
  [ctanThe] -> Product7/2
  [cosPsi] -> Product5/2
  [wy] -> Product3/1
  Product2/1 -> Subtract/2
  Demux/2 -> [wy]
  Product5/1 -> Subtract3/1
  [wy] -> Product5/1
  Integrator3/1 -> [theta3]
  Product6/1 -> Subtract3/2
  Mux/1 -> Out1/1
  Product4/1 -> Subtract1/2
  [theta3] -> Sin/1, Cos1/1
  Product7/1 -> Subtract2/2
  Cos2/1 -> [sinThe]
  Subtract1/1 -> Integrator2/1
  [theta1] -> Mux/1
  Subtract/1 -> Divide1/1
  Demux/3 -> [wz]
  Cos1/1 -> [cosPsi]
  Divide/1 -> [ctanThe]
  In2/1 -> IC/1
  Demux1/2 -> Integrator2/2
  Demux1/3 -> Integrator3/2
  Demux1/1 -> Integrator1/2
  IC/1 -> Demux1/1

== system Lab05/Complete Euler/313To312 ==
  note: Input Interface
  note: Important
      |
      | This system is based on the assumptions that Phi and Psi ranges between [0 and 2*pi] while Theta ranges between [-pi/2 and pi/2]. This is consistent with 312 singularities
  In1 : Inport
  Acos : Trigonometry  Operator=asin
  Acos1 : Trigonometry  Operator=asin
  Atan2 : Trigonometry  Operator=atan2
  Atan3 : Trigonometry  Operator=atan2
  Cos : Trigonometry  Operator=cos
  Cos1 : Trigonometry  Operator=cos
  Cos2 : Trigonometry  Operator=cos
  Demux : Demux  Outputs=3
  Divide{,1..3} (4 alike) : Product  Inputs=*/
  Gain : Gain
  Gain1 : Gain
  Mux : Mux  Inputs=3
  Product{,3,8,11} (4 alike) : Product
  Product4 : Product  Inputs=3
  Product9 : Product  Inputs=3
  Sin : Trigonometry
  Sin1 : Trigonometry
  Sin2 : Trigonometry
  Sin3 : Trigonometry  Operator=cos
  Subtract1 : Sum  Inputs=--
  Subtract3 : Sum  Inputs=-+
  Out1 : Outport
  wires:
  Cos/1 -> [cosPhi313]
  Sin/1 -> [sinPhi313]
  Cos1/1 -> [cosTheta313]
  Demux/3 -> Sin2/1, Cos2/1
  Demux/1 -> Sin/1, Cos/1
  Sin2/1 -> [sinPsi313]
  Sin1/1 -> [sinTheta313]
  In1/1 -> Demux/1
  Demux/2 -> Sin1/1, Cos1/1
  Cos2/1 -> [cosPsi313]
  Mux/1 -> Out1/1
  [sinTheta312] -> Acos/1
  Atan3/1 -> Mux/3
  Atan2/1 -> Mux/1
  [sinPhi312] -> Atan2/1
  [cosPhi312] -> Atan2/2
  [sinPsi312] -> Atan3/1
  [cosPsi312] -> Atan3/2
  Acos/1 -> Mux/2
  [sinTheta313] -> Product/2
  Product/1 -> Acos1/1, [sinTheta312]
  Sin3/1 -> [cosTheta312]
  [cosPsi313] -> Product/1
  Acos1/1 -> Sin3/1
  Gain/1 -> [sinPhi312]
  Divide/1 -> Gain/1
  [cosTheta312] -> Divide/2
  Product3/1 -> Subtract1/1
  [cosPhi313] -> Product3/2
  Product4/1 -> Subtract1/2
  [cosPsi313] -> Product4/1
  [sinPhi313] -> Product4/2
  Subtract1/1 -> Divide/1
  [sinPsi313] -> Product3/1
  [cosTheta313] -> Product4/3
  [cosTheta312] -> Divide1/2
  Divide1/1 -> [cosPhi312]
  [cosPsi313] -> Product9/1
  Product9/1 -> Subtract3/2
  [sinPsi313] -> Product8/1
  [sinPhi313] -> Product8/2
  Product8/1 -> Subtract3/1
  [cosTheta313] -> Product9/3
  Subtract3/1 -> Divide1/1
  [cosPhi313] -> Product9/2
  Divide2/1 -> Gain1/1
  [cosTheta312] -> Divide2/2
  Gain1/1 -> [sinPsi312]
  [sinTheta313] -> Product11/2
  Product11/1 -> Divide2/1
  [sinPsi313] -> Product11/1
  [cosTheta312] -> Divide3/2
  [cosTheta313] -> Divide3/1
  Divide3/1 -> [cosPsi312]

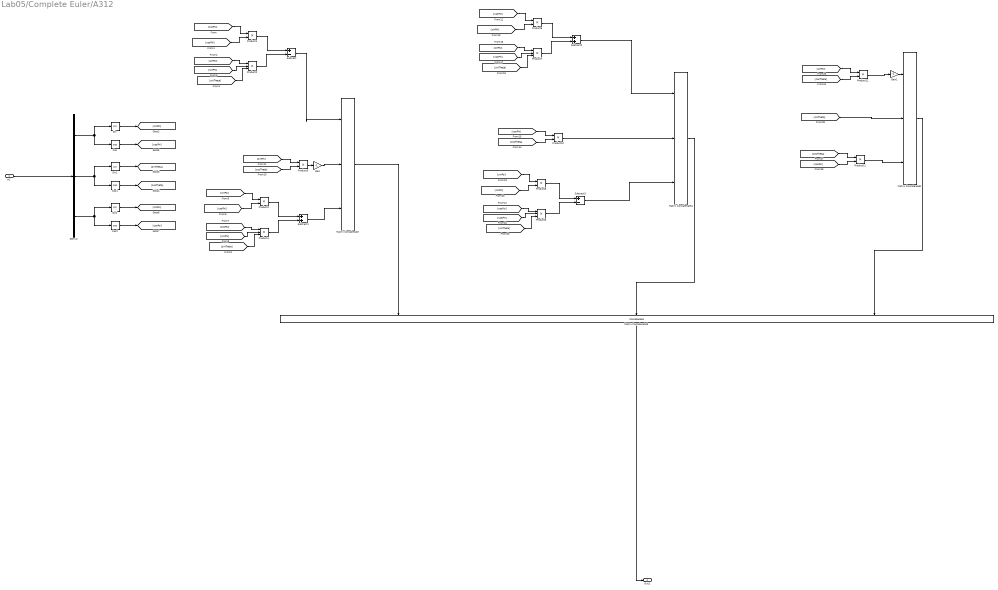
== system Lab05/Complete Euler/A312 ==
  In1 : Inport
  Cos : Trigonometry  Operator=cos
  Cos1 : Trigonometry  Operator=cos
  Cos2 : Trigonometry  Operator=cos
  Demux : Demux  Outputs=3
  Gain : Gain  Gain=-1
  Gain1 : Gain  Gain=-1
  Matrix Concatenate : Concatenate  NumInputs=3  Mode=Multidimensional array
  Matrix Concatenate1 : Concatenate  NumInputs=3  Mode=Multidimensional array
  Matrix Concatenate3 : Concatenate  NumInputs=3  Mode=Multidimensional array  ConcatenateDimension=2
  Matrix Concatenate4 : Concatenate  NumInputs=3  Mode=Multidimensional array
  Product{1,3,5..6,8,10..12} (8 alike) : Product
  Product{2,4,7,9} (4 alike) : Product  Inputs=3
  Sin : Trigonometry
  Sin1 : Trigonometry
  Sin2 : Trigonometry
  Subtract : Sum  Inputs=+-
  Subtract1 : Sum
  Subtract2 : Sum
  Subtract3 : Sum  Inputs=+-
  Out1 : Outport
  wires:
  In1/1 -> Demux/1
  [sinTheta] -> Product2/3
  Product7/1 -> Subtract2/2
  [cosTheta] -> Product11/2
  [sinPhi] -> Product8/2
  Sin/1 -> [sinPhi]
  [sinPhi] -> Product2/2
  [cosTheta] -> Product10/2
  [cosPsi] -> Product6/1
  Demux/3 -> Sin2/1, Cos2/1
  Product9/1 -> Subtract3/2
  [sinTheta] -> Matrix Concatenate1/2
  Matrix Concatenate1/1 -> Matrix Concatenate3/3
  [sinPsi] -> Product11/1
  Product2/1 -> Subtract/2
  Subtract2/1 -> Matrix Concatenate4/1
  Matrix Concatenate4/1 -> Matrix Concatenate3/2
  [cosTheta] -> Product12/1
  Cos2/1 -> [cosPsi]
  [sinPsi] -> Product2/1
  [sinPsi] -> Product8/1
  Sin2/1 -> [sinPsi]
  [sinTheta] -> Product7/3
  Subtract/1 -> Matrix Concatenate/1
  [cosPhi] -> Product10/1
  Demux/2 -> Sin1/1, Cos1/1
  [sinTheta] -> Product9/3
  Product8/1 -> Subtract3/1
  [cosPhi] -> Product9/2
  [cosPsi] -> Product9/1
  Product11/1 -> Gain1/1
  Product1/1 -> Subtract/1
  [cosPhi] -> Product1/2
  [cosPsi] -> Product12/2
  [cosPhi] -> Product7/2
  [sinPhi] -> Product6/2
  Product6/1 -> Subtract2/1
  Demux/1 -> Sin/1, Cos/1
  [cosPsi] -> Product1/1
  [sinPsi] -> Product7/1
  Cos1/1 -> [cosTheta]
  Sin1/1 -> [sinTheta]
  Product12/1 -> Matrix Concatenate1/3
  Matrix Concatenate/1 -> Matrix Concatenate3/1
  Cos/1 -> [cosPhi]
  Matrix Concatenate3/1 -> Out1/1
  Gain1/1 -> Matrix Concatenate1/1
  Product10/1 -> Matrix Concatenate4/2
  Subtract3/1 -> Matrix Concatenate4/3
  [cosPsi] -> Product4/1
  Product4/1 -> Subtract1/2
  [cosPhi] -> Product3/2
  Product3/1 -> Subtract1/1
  [sinPsi] -> Product3/1
  [sinPhi] -> Product4/2
  [sinTheta] -> Product4/3
  [sinPhi] -> Product5/1
  [cosTheta] -> Product5/2
  Product5/1 -> Gain/1
  Subtract1/1 -> Matrix Concatenate/3
  Gain/1 -> Matrix Concatenate/2
